simulink model "gm_sampleModel1573_5_sub"  (R2023a)
settings: Solver=VariableStepAuto  StartTime=0.0  StopTime=10.0  RelTol=1e-3
libraries: simulink x2, hdlsllib x1
settings Model: Creator=user1  LastModifiedBy=user1
settings OptimizationCC: BlockReduction=off  ConditionallyExecuteInputs=off
settings DebuggingCC: InheritedTsInSrcMsg=none

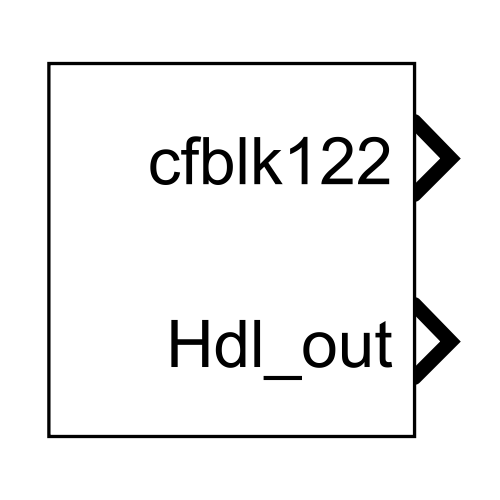
[thumbnail: Simulink's stored preview of the top-level diagram]
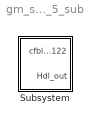
== system gm_sampleModel1573_5_sub ==
  Subsystem : Subsystem

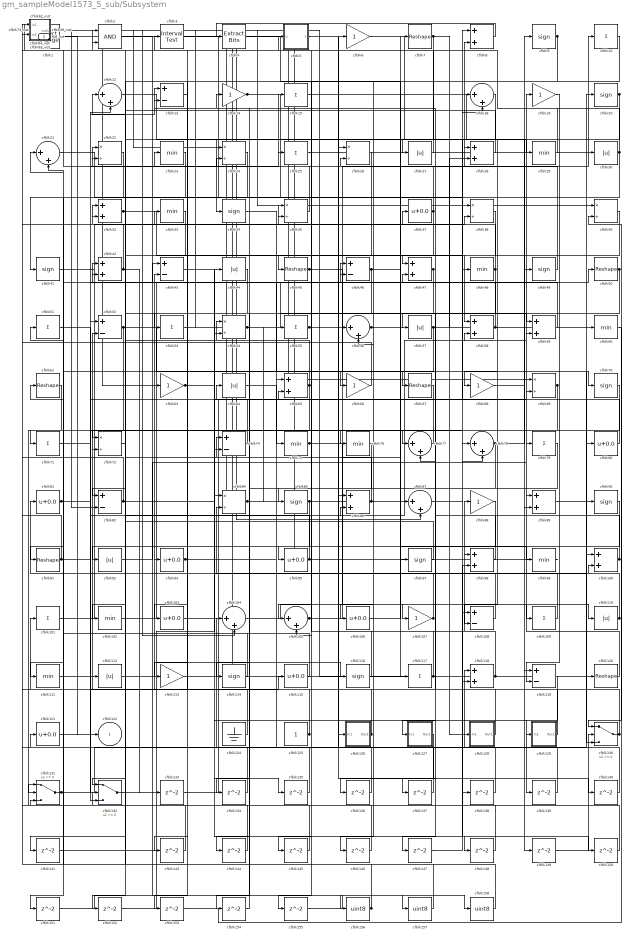
== system gm_sampleModel1573_5_sub/Subsystem ==
  cfblk1 : simulink/Logic and Bit Operations/Detect Change  vinit=0  OutDataTypeStr=uint8
      settings: LibrarySourceBlock=|
      | hdlsllib/Logic and Bit
      | Operations/Detect
      | Change
  cfblk{10,15,25,51,53,55,71,79,101,109,117} (11 alike) : Sum  Inputs=+  OutDataTypeStr=uint8
  cfblk{8,28,32,42,47,58..59,65,86,89,98,100,118} (13 alike) : Sum  OutDataTypeStr=uint8
  cfblk{23,29,33,48,60,75..76,99,102,111} (10 alike) : MinMax  OutDataTypeStr=uint8
  cfblk{37,80..81,93,95,103,106,115,121} (9 alike) : Bias  Bias=0.0  SaturateOnIntegerOverflow=off
  cfblk{12,18,21,56,77..78,87,104..105} (9 alike) : Sum  Inputs=|++  OutDataTypeStr=uint8
  cfblk{6,14,19,63,66,68,88,107,113} (9 alike) : Gain  OutDataTypeStr=uint8
  cfblk{13,43,46,52,74,82,108,119} (8 alike) : Sum  Inputs=+-  OutDataTypeStr=uint8
  cfblk{27,30,44,57,64,92,110,112} (8 alike) : Abs  OutDataTypeStr=uint8  SaturateOnIntegerOverflow=off
  cfblk{9,20,34,41,49,70,85,90,97,114,116} (11 alike) : Signum
  cfblk{7,45,50,61,67,91,120} (7 alike) : Reshape
  cfblk124 : Ground
  cfblk125 : Constant  OutDataTypeStr=uint8  SampleTime=-1
  cfblk126 : Subsystem
  cfblk127 : Subsystem
  cfblk128 : Subsystem
  cfblk129 : Subsystem
  cfblk130 : Switch  OutDataTypeStr=uint8  SaturateOnIntegerOverflow=off  InputSameDT=off
  cfblk131 : Switch  OutDataTypeStr=uint8  SaturateOnIntegerOverflow=off  InputSameDT=off
  cfblk132 : Switch  OutDataTypeStr=uint8  SaturateOnIntegerOverflow=off  InputSameDT=off
  cfblk{133..141,143..155} (22 alike) : Delay  SampleTime=1
  cfblk156 : DataTypeConversion  OutDataTypeStr=uint8  SaturateOnIntegerOverflow=off  RndMeth=Floor
  cfblk157 : DataTypeConversion  OutDataTypeStr=uint8  SaturateOnIntegerOverflow=off  RndMeth=Floor
  cfblk158 : DataTypeConversion  OutDataTypeStr=uint8  SaturateOnIntegerOverflow=off  RndMeth=Floor
  cfblk16_inst : Subsystem
  cfblk17_inst : Subsystem
  cfblk2 : Logic  AllPortsSameDT=off  OutDataTypeStr=boolean
  cfblk{22,24,26,35,38,40,54,69,72,84} (10 alike) : Product  Inputs=*/  OutDataTypeStr=uint8  RndMeth=Zero  SaturateOnIntegerOverflow=on
  cfblk3 : hdlsllib/Logic and Bit Operations/Interval Test  IntervalClosedRight=on  uplimit=0.5  IntervalClosedLeft=on  lowlimit=-0.5  OutDataTypeStr=uint8
  cfblk31_inst : Subsystem
  cfblk36_inst : Subsystem
  cfblk39_inst : Subsystem
  cfblk4 : simulink/Logic and Bit Operations/Extract Bits  bitsToExtract=Upper half  numBits=8  bitIdxRange=[0 7]  outScalingMode=Preserve fixed-point scaling
      settings: LibrarySourceBlock=|
      | hdlsllib/Logic and Bit
      | Operations/Extract Bits
  cfblk5 : Subsystem  mask(Detect Rise Nonnegative){vinit=double(0), InputProcessing=Elements as channels (sample based), OutDataTypeStr=uint8}
      mask prompts: vinit "Simulink:masks:InitialCondition_MP"; InputProcessing "Simulink:masks:InputProcessing_MP"; OutDataTypeStr "Simulink:masks:OutputDataType_MP"
      mask help: Simulink:masks:DetectRiseNonnegative_MD
      mask init:
      | InputProcessing = 'Elements as channels (sample based)';
      | OutDataTypeStr = 'uint8';
      | vinit = double(0);
      mask TypeOptions InputProcessing: Simulink:masks:ColumnsAsChannelsFrameBased | Simulink:masks:ElementsAsChannelsSampleBased
      mask TypeOptions OutDataTypeStr: Simulink:masks:uint8 | Simulink:masks:boolean
      mask Display: fprintf('U >= 0\n&  NOT\nU/z >= 0')
  cfblk62_inst : Subsystem
  cfblk73_inst : Subsystem
  cfblk83_inst : Subsystem
  cfblk94_inst : Subsystem
  cfblk122 : Outport  OutDataTypeStr=uint8  SampleTime=1  VectorParamsAs1DForOutWhenUnconnected=off
  Hdl_out : Outport  Port=2  OutDataTypeStr=uint8  SampleTime=1
  wires:
  cfblk1/1 -> cfblk122/1
  cfblk10/1 -> cfblk141/1
  cfblk100/1 -> cfblk47/2, cfblk32/1, cfblk26/2
  cfblk101/1 -> cfblk35/1
  cfblk102/1 -> cfblk50/1
  cfblk103/1 -> cfblk65/2
  cfblk104/1 -> cfblk107/1
  cfblk105/1 -> cfblk8/2, cfblk10/1
  cfblk106/1 -> cfblk28/1
  cfblk107/1 -> cfblk43/2, cfblk84/2
  cfblk108/1 -> cfblk81/1
  cfblk109/1 -> cfblk88/1
  cfblk110/1 -> cfblk100/2, cfblk19/1
  cfblk111/1 -> cfblk52/2
  cfblk112/1 -> cfblk116/1
  cfblk113/1 -> cfblk6/1
  cfblk114/1 -> cfblk23/1
  cfblk115/1 -> cfblk61/1
  cfblk116/1 -> cfblk64/1
  cfblk117/1 -> cfblk39_inst/1(in1), Hdl_out/1
  cfblk118/1 -> cfblk98/1, cfblk16_inst/2(in2)
  cfblk119/1 -> cfblk139/1
  cfblk12/1 -> cfblk138/1
  cfblk120/1 -> cfblk89/1
  cfblk121/1 -> cfblk115/1
  cfblk124/1 -> cfblk101/1
  cfblk125/1 -> cfblk74/1, cfblk72/2
  cfblk126/1(Out1) -> cfblk93/1, cfblk112/1
  cfblk127/1(Out1) -> cfblk136/1
  cfblk128/1(Out1) -> cfblk51/1
  cfblk129/1(Out1) -> cfblk3/1
  cfblk13/1 -> cfblk103/1
  cfblk130/1 -> cfblk83_inst/2(in2), cfblk77/2
  cfblk131/1 -> cfblk20/1, cfblk12/2
  cfblk132/1 -> cfblk44/1
  cfblk133/1 -> cfblk58/2
  cfblk134/1 -> cfblk104/1
  cfblk135/1 -> cfblk65/1
  cfblk136/1 -> cfblk39_inst/2(in2)
  cfblk137/1 -> cfblk21/2
  cfblk138/1 -> cfblk17_inst/2(in2)
  cfblk139/1 -> cfblk118/1
  cfblk14/1 -> cfblk27/1, cfblk126/1(In1)
  cfblk140/1 -> cfblk26/1
  cfblk141/1 -> cfblk100/1
  cfblk143/1 -> cfblk73_inst/2(in2)
  cfblk144/1 -> cfblk131/3
  cfblk145/1 -> cfblk94_inst/1(in1)
  cfblk146/1 -> cfblk131/1
  cfblk147/1 -> cfblk98/2
  cfblk148/1 -> cfblk132/2
  cfblk149/1 -> cfblk130/2
  cfblk15/1 -> cfblk29/1
  cfblk150/1 -> cfblk83_inst/1(in1)
  cfblk151/1 -> cfblk157/1
  cfblk152/1 -> cfblk84/1
  cfblk153/1 -> cfblk40/2
  cfblk154/1 -> cfblk54/1
  cfblk155/1 -> cfblk158/1
  cfblk156/1 -> cfblk17_inst/1(in1), cfblk121/1
  cfblk157/1 -> cfblk2/1
  cfblk158/1 -> cfblk2/2
  cfblk16_inst/1(out1) -> cfblk18/1, cfblk38/1, cfblk60/1
  cfblk17_inst/1(out1) -> cfblk40/1
  cfblk18/1 -> cfblk152/1
  cfblk19/1 -> cfblk119/2
  cfblk2/1 -> cfblk156/1
  cfblk20/1 -> cfblk34/1, cfblk108/2
  cfblk21/1 -> cfblk117/1
  cfblk22/1 -> cfblk111/1
  cfblk23/1 -> cfblk91/1
  cfblk24/1 -> cfblk41/1
  cfblk25/1 -> cfblk140/1
  cfblk26/1 -> cfblk132/1
  cfblk27/1 -> cfblk36_inst/2(in2)
  cfblk28/1 -> cfblk94_inst/2(in2)
  cfblk29/1 -> cfblk62_inst/1(in1)
  cfblk3/1 -> cfblk108/1
  cfblk30/1 -> cfblk82/1, cfblk31_inst/2(in2), cfblk68/1
  cfblk31_inst/1(out1) -> cfblk69/1
  cfblk32/1 -> cfblk78/1, cfblk35/2
  cfblk33/1 -> cfblk72/1
  cfblk34/1 -> cfblk66/1
  cfblk35/1 -> cfblk15/1
  cfblk36_inst/1(out1) -> cfblk63/1
  cfblk37/1 -> cfblk73_inst/1(in1), cfblk113/1
  cfblk38/1 -> cfblk45/1
  cfblk39_inst/1(out1) -> cfblk82/2, cfblk24/1
  cfblk4/1 -> cfblk97/1
  cfblk40/1 -> cfblk58/1
  cfblk41/1 -> cfblk37/1
  cfblk42/1 -> cfblk62_inst/2(in2), cfblk133/1
  cfblk43/1 -> cfblk135/1
  cfblk44/1 -> cfblk92/1
  cfblk45/1 -> cfblk57/1, cfblk130/3
  cfblk46/1 -> cfblk70/1, cfblk144/1
  cfblk47/1 -> cfblk146/1, cfblk145/1
  cfblk48/1 -> cfblk137/1, cfblk33/1
  cfblk49/1 -> cfblk5/1(U)
  cfblk5/1(Y) -> cfblk47/1
  cfblk50/1 -> cfblk54/2, cfblk155/1
  cfblk51/1 -> cfblk78/2
  cfblk52/1 -> cfblk89/2, cfblk132/3
  cfblk53/1 -> cfblk67/1
  cfblk54/1 -> cfblk9/1, cfblk59/1
  cfblk55/1 -> cfblk80/1, cfblk8/1, cfblk118/2
  cfblk56/1 -> cfblk106/1, cfblk99/1
  cfblk57/1 -> cfblk59/2, cfblk28/2, cfblk18/2, cfblk151/1
  cfblk58/1 -> cfblk21/1, cfblk24/2
  cfblk59/1 -> cfblk43/1
  cfblk6/1 -> cfblk119/1
  cfblk60/1 -> cfblk130/1
  cfblk61/1 -> cfblk71/1
  cfblk62_inst/1(out1) -> cfblk120/1
  cfblk63/1 -> cfblk148/1, cfblk129/1(In1)
  cfblk64/1 -> cfblk75/1
  cfblk65/1 -> cfblk85/1, cfblk74/2, cfblk22/1
  cfblk66/1 -> cfblk36_inst/1(in1)
  cfblk67/1 -> cfblk154/1
  cfblk68/1 -> cfblk149/1
  cfblk69/1 -> cfblk131/2, cfblk143/1
  cfblk7/1 -> cfblk105/2, cfblk128/1(In1)
  cfblk70/1 -> cfblk77/1
  cfblk71/1 -> cfblk13/1
  cfblk72/1 -> cfblk12/1
  cfblk73_inst/1(out1) -> cfblk104/2
  cfblk74/1 -> cfblk52/1
  cfblk75/1 -> cfblk110/1, cfblk109/1, cfblk48/1
  cfblk76/1 -> cfblk105/1
  cfblk77/1 -> cfblk76/1
  cfblk78/1 -> cfblk49/1, cfblk147/1
  cfblk79/1 -> cfblk114/1
  cfblk8/1 -> cfblk4/1
  cfblk80/1 -> cfblk42/1
  cfblk81/1 -> cfblk86/2, cfblk46/1
  cfblk82/1 -> cfblk31_inst/1(in1), cfblk69/2
  cfblk83_inst/1(out1) -> cfblk87/2, cfblk56/1
  cfblk84/1 -> cfblk46/2, cfblk55/1
  cfblk85/1 -> cfblk38/2, cfblk102/1
  cfblk86/1 -> cfblk7/1, cfblk32/2
  cfblk87/1 -> cfblk150/1
  cfblk88/1 -> cfblk127/1(In1)
  cfblk89/1 -> cfblk90/1
  cfblk9/1 -> cfblk95/1, cfblk56/2, cfblk53/1
  cfblk90/1 -> cfblk134/1
  cfblk91/1 -> cfblk16_inst/1(in1), cfblk25/1
  cfblk92/1 -> cfblk79/1
  cfblk93/1 -> cfblk86/1, cfblk153/1
  cfblk94_inst/1(out1) -> cfblk87/1, cfblk30/1
  cfblk95/1 -> cfblk22/2, cfblk14/1
  cfblk97/1 -> cfblk42/2
  cfblk98/1 -> cfblk13/2
  cfblk99/1 -> cfblk1/1

== system gm_sampleModel1573_5_sub/Subsystem/cfblk126 ==
  In1 : Inport  OutDataTypeStr=uint8  PortDimensions=1  SampleTime=1
  Out1 : Outport  SampleTime=1
  wires:
  In1/1 -> Out1/1

== system gm_sampleModel1573_5_sub/Subsystem/cfblk127 ==
  In1 : Inport  OutDataTypeStr=uint8  PortDimensions=1  SampleTime=1
  Out1 : Outport  SampleTime=1
  wires:
  In1/1 -> Out1/1

== system gm_sampleModel1573_5_sub/Subsystem/cfblk128 ==
  In1 : Inport  OutDataTypeStr=uint8  PortDimensions=1  SampleTime=1
  Out1 : Outport  SampleTime=1
  wires:
  In1/1 -> Out1/1

== system gm_sampleModel1573_5_sub/Subsystem/cfblk129 ==
  In1 : Inport  OutDataTypeStr=uint8  PortDimensions=1  SampleTime=1
  Out1 : Outport  SampleTime=1
  wires:
  In1/1 -> Out1/1

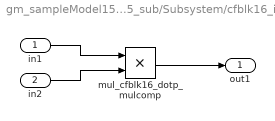
== system gm_sampleModel1573_5_sub/Subsystem/cfblk16_inst ==
  in1 : Inport  OutDataTypeStr=uint8  SampleTime=1
  in2 : Inport  Port=2  OutDataTypeStr=uint8  SampleTime=1
  mul_cfblk16_dotp_mulcomp : Product  Inputs=**  OutDataTypeStr=uint8  SampleTime=1
  out1 : Outport  OutDataTypeStr=uint8  SampleTime=1
  wires:
  in1/1 -> mul_cfblk16_dotp_mulcomp/1
  in2/1 -> mul_cfblk16_dotp_mulcomp/2
  mul_cfblk16_dotp_mulcomp/1 -> out1/1

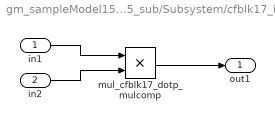
== system gm_sampleModel1573_5_sub/Subsystem/cfblk17_inst ==
  in1 : Inport  OutDataTypeStr=uint8  SampleTime=1
  in2 : Inport  Port=2  OutDataTypeStr=uint8  SampleTime=1
  mul_cfblk17_dotp_mulcomp : Product  Inputs=**  OutDataTypeStr=uint8  SampleTime=1
  out1 : Outport  OutDataTypeStr=uint8  SampleTime=1
  wires:
  in1/1 -> mul_cfblk17_dotp_mulcomp/1
  in2/1 -> mul_cfblk17_dotp_mulcomp/2
  mul_cfblk17_dotp_mulcomp/1 -> out1/1

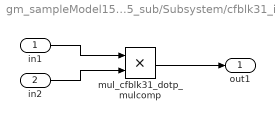
== system gm_sampleModel1573_5_sub/Subsystem/cfblk31_inst ==
  in1 : Inport  OutDataTypeStr=uint8  SampleTime=1
  in2 : Inport  Port=2  OutDataTypeStr=uint8  SampleTime=1
  mul_cfblk31_dotp_mulcomp : Product  Inputs=**  OutDataTypeStr=uint8  SampleTime=1
  out1 : Outport  OutDataTypeStr=uint8  SampleTime=1
  wires:
  in1/1 -> mul_cfblk31_dotp_mulcomp/1
  in2/1 -> mul_cfblk31_dotp_mulcomp/2
  mul_cfblk31_dotp_mulcomp/1 -> out1/1

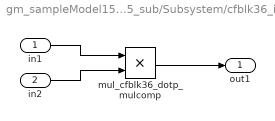
== system gm_sampleModel1573_5_sub/Subsystem/cfblk36_inst ==
  in1 : Inport  OutDataTypeStr=uint8  SampleTime=1
  in2 : Inport  Port=2  OutDataTypeStr=uint8  SampleTime=1
  mul_cfblk36_dotp_mulcomp : Product  Inputs=**  OutDataTypeStr=uint8  SampleTime=1
  out1 : Outport  OutDataTypeStr=uint8  SampleTime=1
  wires:
  in1/1 -> mul_cfblk36_dotp_mulcomp/1
  in2/1 -> mul_cfblk36_dotp_mulcomp/2
  mul_cfblk36_dotp_mulcomp/1 -> out1/1

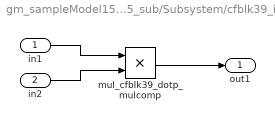
== system gm_sampleModel1573_5_sub/Subsystem/cfblk39_inst ==
  in1 : Inport  OutDataTypeStr=uint8  SampleTime=1
  in2 : Inport  Port=2  OutDataTypeStr=uint8  SampleTime=1
  mul_cfblk39_dotp_mulcomp : Product  Inputs=**  OutDataTypeStr=uint8  SampleTime=1
  out1 : Outport  OutDataTypeStr=uint8  SampleTime=1
  wires:
  in1/1 -> mul_cfblk39_dotp_mulcomp/1
  in2/1 -> mul_cfblk39_dotp_mulcomp/2
  mul_cfblk39_dotp_mulcomp/1 -> out1/1

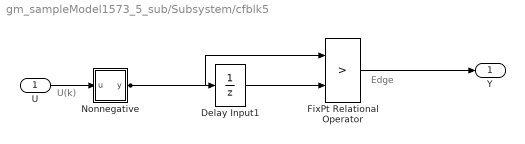
== system gm_sampleModel1573_5_sub/Subsystem/cfblk5 ==
  note: U(k)
  note: Edge
  U : Inport  OutDataTypeStr=uint8  SampleTime=1
  Delay Input1 : UnitDelay  Description=Store in Global RAM  DisableCoverage=on  InitialCondition=vinit  SampleTime=-1  HasFrameUpgradeWarning=on
  FixPt Relational Operator : RelationalOperator  Operator=>  OutDataTypeStr=fixdt(0, 8)  ZeroCross=off  InputSameDT=off
  Nonnegative : Subsystem  mask(Compare To Zero){relop=>=, OutDataTypeStr=boolean, ZeroCross=off}
      mask prompts: relop "Simulink:masks:Operator_MP"; OutDataTypeStr "Simulink:masks:OutputDataType_MP"; ZeroCross "Simulink:masks:EnableZerocrossingDetection_MP"
      mask help: Simulink:masks:CompareToZero_MD
      mask init:
      | OutDataTypeStr = 'boolean';
      | ZeroCross = 'off';
      | blkName = 'sampleModel1573_5_sub/Subsystem/cfblk5/Nonnegative';
      | relop = '>=';
      | setValue = 'boolean';
      mask TypeOptions relop: == | ~= | < | <= | >= | >
      mask TypeOptions OutDataTypeStr: Simulink:masks:uint8 | Simulink:masks:boolean
      mask Callback ZeroCross: sl('zeroCrossEnable', gcbh);
      mask Display: disp([relop,' 0'])
  Y : Outport  SampleTime=1
  wires:
  U/1 -> Nonnegative/1(u)
  Delay Input1/1 -> FixPt Relational Operator/2
  FixPt Relational Operator/1 -> Y/1
  Nonnegative/1(y) -> FixPt Relational Operator/1, Delay Input1/1

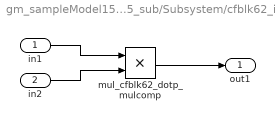
== system gm_sampleModel1573_5_sub/Subsystem/cfblk62_inst ==
  in1 : Inport  OutDataTypeStr=uint8  SampleTime=1
  in2 : Inport  Port=2  OutDataTypeStr=uint8  SampleTime=1
  mul_cfblk62_dotp_mulcomp : Product  Inputs=**  OutDataTypeStr=uint8  SampleTime=1
  out1 : Outport  OutDataTypeStr=uint8  SampleTime=1
  wires:
  in1/1 -> mul_cfblk62_dotp_mulcomp/1
  in2/1 -> mul_cfblk62_dotp_mulcomp/2
  mul_cfblk62_dotp_mulcomp/1 -> out1/1

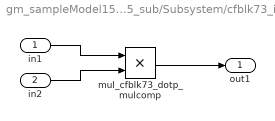
== system gm_sampleModel1573_5_sub/Subsystem/cfblk73_inst ==
  in1 : Inport  OutDataTypeStr=uint8  SampleTime=1
  in2 : Inport  Port=2  OutDataTypeStr=uint8  SampleTime=1
  mul_cfblk73_dotp_mulcomp : Product  Inputs=**  OutDataTypeStr=uint8  SampleTime=1
  out1 : Outport  OutDataTypeStr=uint8  SampleTime=1
  wires:
  in1/1 -> mul_cfblk73_dotp_mulcomp/1
  in2/1 -> mul_cfblk73_dotp_mulcomp/2
  mul_cfblk73_dotp_mulcomp/1 -> out1/1

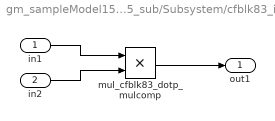
== system gm_sampleModel1573_5_sub/Subsystem/cfblk83_inst ==
  in1 : Inport  OutDataTypeStr=uint8  SampleTime=1
  in2 : Inport  Port=2  OutDataTypeStr=uint8  SampleTime=1
  mul_cfblk83_dotp_mulcomp : Product  Inputs=**  OutDataTypeStr=uint8  SampleTime=1
  out1 : Outport  OutDataTypeStr=uint8  SampleTime=1
  wires:
  in1/1 -> mul_cfblk83_dotp_mulcomp/1
  in2/1 -> mul_cfblk83_dotp_mulcomp/2
  mul_cfblk83_dotp_mulcomp/1 -> out1/1

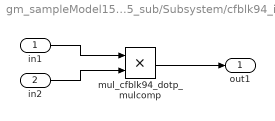
== system gm_sampleModel1573_5_sub/Subsystem/cfblk94_inst ==
  in1 : Inport  OutDataTypeStr=uint8  SampleTime=1
  in2 : Inport  Port=2  OutDataTypeStr=uint8  SampleTime=1
  mul_cfblk94_dotp_mulcomp : Product  Inputs=**  OutDataTypeStr=uint8  SampleTime=1
  out1 : Outport  OutDataTypeStr=uint8  SampleTime=1
  wires:
  in1/1 -> mul_cfblk94_dotp_mulcomp/1
  in2/1 -> mul_cfblk94_dotp_mulcomp/2
  mul_cfblk94_dotp_mulcomp/1 -> out1/1

== system gm_sampleModel1573_5_sub/Subsystem/cfblk5/Nonnegative ==
  u : Inport  OutDataTypeStr=uint8  SampleTime=1
  Compare : RelationalOperator  OutDataTypeStr=boolean  ZeroCross=off
  Constant : Constant  DisableCoverage=on  Value=0  OutDataTypeStr=Inherit: Inherit via back propagation  SampleTime=-1  PreserveConstantTs=on
  y : Outport  SampleTime=1
  wires:
  u/1 -> Compare/1
  Compare/1 -> y/1
  Constant/1 -> Compare/2
